simulink model "Thesis_MMC_WF_Modify"  (R2023a)
settings: Solver=VariableStepAuto  StartTime=0.0  StopTime=16  RelTol=1e-3
InitFcn:
  | % TS %
  | Ts_Control=4e-05;
  | Ts_Power=2e-05;
  | %% Main Circuit %%
  | % AC Line %
  | Vnom_Sec=333000;
  | Vnom_Pri=400000;
  | Pnom=1.0e+09;
  | Fnom=60;
  | Psc=2.0e+10;
  | P_Ld1=2/3*1e+09;
  | R_Startup=400;
  | Rxfo=0.003;
  | Lxfo=0.12;
  | P_Ld2=500e+03;
  | % MMC Parameter %
  | Larm_pu=0.15;
  | Rarm_pu=Larm_pu/100;
  | Zbase= Vnom_Sec^2/Pnom;
  | Larm=Larm_pu*(Zbase/(2*pi*Fnom));
  | Rarm=Rarm_pu*Zbase;
  | C_PM=1.758e-3;
  | w=2*pi*Fnom;
  | wc2=(2*w)^2;
  | Cfilter=1/(Larm*wc2);
  | Rfilter=1/(Cfilter*w)*30;
  | Topen_Filter=1e6;
  | K_V_dc=600000;
  | n=36;
  | Rg=100;
  | Cg=5e-08;
  | % HVDC Parameter %
  | R_cable=0.5;
  | L_cable=0.015;
  | %% Controller Parameter %%
  | % PLL %
  | Fn_filter=1000;
  | Zeta_filter=1;
  | % Active Power Regulator %
  | Kp_Preg=1/6;
  | Ki_Preg=1;
  | Limits_Preg=[0.8 1.2];
  | set_param('Thesis_MMC_WF_Modify/Controller/Active Power Regulator/Sum1','SampleTime','Ts_Control')
  | set_param('Thesis_MMC_WF_Modify/Controller/Active Power Regulator/Saturation','SampleTime','Ts_Control')
  | % Reactive Power Regulator %
  | Kp_Qreg=1/6;
  | Ki_Qreg=1;
  | Limits_Qreg=[-0.25 0.25];
  | set_param('Thesis_MMC_WF_Modify/Controller/Reactive Power Regulartor/Sum1','SampleTime','Ts_Control')
  | % Discrete Mean %
  | K1=3.2312e-30;
  | K2=-1.1369e-16;
  | Delay=0.02;
  | Vint=0;
  | Delay1=0.02004;
  | % DC Voltage Regulator %
  | Kp_VDCreg=4;
  | Ki_VDCreg=100;
  | Limits_VDCreg=[-2 2];
  | set_param('Thesis_MMC_WF_Modify/Controller/DC Voltage Regulator/Sum1','SampleTime','Ts_Control')
  | ... (+46 lines)
undefined symbols (not defined in the file): D1, Delta, Delta1, DiscIntNeverNeededParam, Lagging, Vnom_dc
libraries: spsSeriesRLCBranchLib x54, spsIGBTLib x24, spsBreakerLib x13, spsVoltageMeasurementLib x11, spsThreePhaseBreakerLib x11, spsThreePhaseVIMeasurementLib x9, spsIdealSwitchLib x8, simulink x7, spsDiscreteVariableTimeDelayLib x7, spsCurrentMeasurementLib x6, spsGroundLib x6, spsSecondOrderFilterLib x6
(part 2 of 3)

== system Thesis_MMC_WF_Modify/Inverter1 ==
  Constant6 : Constant  Value=480000/2  SampleTime=Ts_Power
  Controlled Voltage Source : spsControlledVoltageSourceLib/Controlled Voltage Source  Initialize=off  Source_Type=DC  Amplitude=0  Phase=0  Frequency=0  Measurements=None
  Controlled Voltage Source4 : spsControlledVoltageSourceLib/Controlled Voltage Source  Initialize=off  Source_Type=DC  Amplitude=0  Phase=0  Frequency=0  Measurements=None
  Ground : spsGroundLib/Ground  LConnTagsString=a
  Ideal Switch : spsIdealSwitchLib/Ideal Switch  Ron=0.001  Lon=0  IC=0  Rs=1e6  Cs=inf  Measurements=off
  Ideal Switch1 : spsIdealSwitchLib/Ideal Switch  Ron=0.001  Lon=0  IC=0  Rs=1e6  Cs=inf  Measurements=off
  Series RLC Branch : spsSeriesRLCBranchLib/Series RLC Branch  LConnTagsString=__new0  RConnTagsString=__new0  BranchType=RC  Resistance=1e-3  Inductance=1e-3  SetiL0=off  InitialCurrent=0  Capacitance=C_PM/n*3  Setx0=off  InitialVoltage=0  Measurements=None
  Series RLC Branch1 : spsSeriesRLCBranchLib/Series RLC Branch  LConnTagsString=__new0  RConnTagsString=__new0  BranchType=RC  Resistance=1e-3  Inductance=1e-3  SetiL0=off  InitialCurrent=0  Capacitance=C_PM/n*3  Setx0=off  InitialVoltage=0  Measurements=None
  Series RLC Branch2 : spsSeriesRLCBranchLib/Series RLC Branch  LConnTagsString=__new0  RConnTagsString=__new0  BranchType=R  Resistance=1e-3  Inductance=1e-3  SetiL0=off  InitialCurrent=0  Capacitance=1e-6  Setx0=off  InitialVoltage=0  Measurements=None
  Series RLC Branch3 : spsSeriesRLCBranchLib/Series RLC Branch  LConnTagsString=__new0  RConnTagsString=__new0  BranchType=R  Resistance=1e-3  Inductance=1e-3  SetiL0=off  InitialCurrent=0  Capacitance=1e-6  Setx0=off  InitialVoltage=0  Measurements=None
  Series RLC Branch5 : spsSeriesRLCBranchLib/Series RLC Branch  LConnTagsString=__new0  RConnTagsString=__new0  BranchType=RL  Resistance=1e-2  Inductance=1e-4  SetiL0=off  InitialCurrent=0  Capacitance=1e-6  Setx0=off  InitialVoltage=0  Measurements=None
  Series RLC Branch6 : spsSeriesRLCBranchLib/Series RLC Branch  LConnTagsString=__new0  RConnTagsString=__new0  BranchType=RL  Resistance=1e-2  Inductance=1e-4  SetiL0=off  InitialCurrent=0  Capacitance=1e-6  Setx0=off  InitialVoltage=0  Measurements=None
  Voltage Measurement1 : spsVoltageMeasurementLib/Voltage Measurement  PhasorSimulation=off  OutputType=Complex  PSBequivalent=0
  1 : PMIOPort  Side=Left
  2 : PMIOPort  Port=2  Side=Left
  tag scope: Vdc2=global
  wires:
  Constant6/1 -> Controlled Voltage Source/1, Controlled Voltage Source4/1
  [Inverter1_On] -> Ideal Switch/1, Ideal Switch1/1
  Voltage Measurement1/1 -> [Vdc2]
  connections:
  2/RConn1 -- Voltage Measurement1/LConn2 -- Series RLC Branch3/LConn1 -- Series RLC Branch1/RConn1
  Ideal Switch1/RConn1 -- Series RLC Branch6/RConn1
  Controlled Voltage Source4/RConn1 -- Controlled Voltage Source/LConn1 -- Series RLC Branch1/LConn1 -- Series RLC Branch/RConn1 -- Ground/LConn1
  Ideal Switch/RConn1 -- Series RLC Branch5/LConn1
  1/RConn1 -- Voltage Measurement1/LConn1 -- Series RLC Branch2/LConn1 -- Series RLC Branch/LConn1
  Series RLC Branch3/RConn1 -- Ideal Switch1/LConn1
  Series RLC Branch2/RConn1 -- Ideal Switch/LConn1
  Controlled Voltage Source/RConn1 -- Series RLC Branch5/RConn1
  Controlled Voltage Source4/LConn1 -- Series RLC Branch6/LConn1

== system Thesis_MMC_WF_Modify/Inverter2 ==
  Constant6 : Constant  Value=640000/2  SampleTime=Ts_Power
  Controlled Voltage Source : spsControlledVoltageSourceLib/Controlled Voltage Source  Initialize=off  Source_Type=DC  Amplitude=0  Phase=0  Frequency=0  Measurements=None
  Controlled Voltage Source4 : spsControlledVoltageSourceLib/Controlled Voltage Source  Initialize=off  Source_Type=DC  Amplitude=0  Phase=0  Frequency=0  Measurements=None
  Ground : spsGroundLib/Ground  LConnTagsString=a
  Ideal Switch : spsIdealSwitchLib/Ideal Switch  Ron=0.001  Lon=0  IC=0  Rs=1e6  Cs=inf  Measurements=off
  Ideal Switch1 : spsIdealSwitchLib/Ideal Switch  Ron=0.001  Lon=0  IC=0  Rs=1e6  Cs=inf  Measurements=off
  Series RLC Branch : spsSeriesRLCBranchLib/Series RLC Branch  LConnTagsString=__new0  RConnTagsString=__new0  BranchType=RC  Resistance=1e-3  Inductance=1e-3  SetiL0=off  InitialCurrent=0  Capacitance=C_PM/n*3  Setx0=off  InitialVoltage=0  Measurements=None
  Series RLC Branch1 : spsSeriesRLCBranchLib/Series RLC Branch  LConnTagsString=__new0  RConnTagsString=__new0  BranchType=RC  Resistance=1e-3  Inductance=1e-3  SetiL0=off  InitialCurrent=0  Capacitance=C_PM/n*3  Setx0=off  InitialVoltage=0  Measurements=None
  Series RLC Branch2 : spsSeriesRLCBranchLib/Series RLC Branch  LConnTagsString=__new0  RConnTagsString=__new0  BranchType=R  Resistance=1e-3  Inductance=1e-3  SetiL0=off  InitialCurrent=0  Capacitance=1e-6  Setx0=off  InitialVoltage=0  Measurements=None
  Series RLC Branch3 : spsSeriesRLCBranchLib/Series RLC Branch  LConnTagsString=__new0  RConnTagsString=__new0  BranchType=R  Resistance=1e-3  Inductance=1e-3  SetiL0=off  InitialCurrent=0  Capacitance=1e-6  Setx0=off  InitialVoltage=0  Measurements=None
  Series RLC Branch5 : spsSeriesRLCBranchLib/Series RLC Branch  LConnTagsString=__new0  RConnTagsString=__new0  BranchType=RL  Resistance=1e-2  Inductance=1e-4  SetiL0=off  InitialCurrent=0  Capacitance=1e-6  Setx0=off  InitialVoltage=0  Measurements=None
  Series RLC Branch6 : spsSeriesRLCBranchLib/Series RLC Branch  LConnTagsString=__new0  RConnTagsString=__new0  BranchType=RL  Resistance=1e-2  Inductance=1e-4  SetiL0=off  InitialCurrent=0  Capacitance=1e-6  Setx0=off  InitialVoltage=0  Measurements=None
  Voltage Measurement1 : spsVoltageMeasurementLib/Voltage Measurement  PhasorSimulation=off  OutputType=Complex  PSBequivalent=0
  1 : PMIOPort  Side=Left
  2 : PMIOPort  Port=2  Side=Left
  tag scope: Vdc4=global
  wires:
  Constant6/1 -> Controlled Voltage Source/1, Controlled Voltage Source4/1
  [Inverter2_On] -> Ideal Switch/1, Ideal Switch1/1
  Voltage Measurement1/1 -> [Vdc4]
  connections:
  2/RConn1 -- Voltage Measurement1/LConn2 -- Series RLC Branch3/LConn1 -- Series RLC Branch1/RConn1
  Ideal Switch1/RConn1 -- Series RLC Branch6/RConn1
  Series RLC Branch/RConn1 -- Ground/LConn1 -- Controlled Voltage Source/LConn1 -- Controlled Voltage Source4/RConn1 -- Series RLC Branch1/LConn1
  Ideal Switch/RConn1 -- Series RLC Branch5/LConn1
  1/RConn1 -- Voltage Measurement1/LConn1 -- Series RLC Branch2/LConn1 -- Series RLC Branch/LConn1
  Series RLC Branch3/RConn1 -- Ideal Switch1/LConn1
  Series RLC Branch2/RConn1 -- Ideal Switch/LConn1
  Controlled Voltage Source/RConn1 -- Series RLC Branch5/RConn1
  Controlled Voltage Source4/LConn1 -- Series RLC Branch6/LConn1

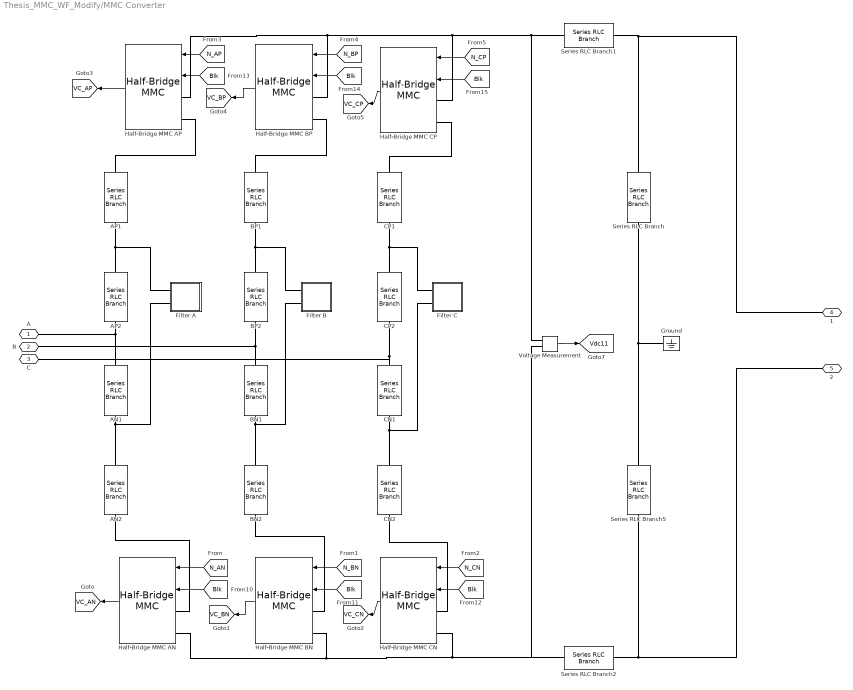
== system Thesis_MMC_WF_Modify/MMC Converter ==
  AN1 : spsSeriesRLCBranchLib/Series RLC Branch  LConnTagsString=__new0  RConnTagsString=__new0  BranchType=RL  Resistance=Rarm/2  Inductance=Larm/2  SetiL0=off  InitialCurrent=0  Capacitance=1e-6  Setx0=off  InitialVoltage=0  Measurements=None
  AN2 : spsSeriesRLCBranchLib/Series RLC Branch  LConnTagsString=__new0  RConnTagsString=__new0  BranchType=RL  Resistance=Rarm/2  Inductance=Larm/2  SetiL0=off  InitialCurrent=0  Capacitance=1e-6  Setx0=off  InitialVoltage=0  Measurements=None
  AP1 : spsSeriesRLCBranchLib/Series RLC Branch  LConnTagsString=__new0  RConnTagsString=__new0  BranchType=RL  Resistance=Rarm/2  Inductance=Larm/2  SetiL0=off  InitialCurrent=0  Capacitance=1e-6  Setx0=off  InitialVoltage=0  Measurements=None
  AP2 : spsSeriesRLCBranchLib/Series RLC Branch  LConnTagsString=__new0  RConnTagsString=__new0  BranchType=RL  Resistance=Rarm/2  Inductance=Larm/2  SetiL0=off  InitialCurrent=0  Capacitance=1e-6  Setx0=off  InitialVoltage=0  Measurements=None
  BN1 : spsSeriesRLCBranchLib/Series RLC Branch  LConnTagsString=__new0  RConnTagsString=__new0  BranchType=RL  Resistance=Rarm/2  Inductance=Larm/2  SetiL0=off  InitialCurrent=0  Capacitance=1e-6  Setx0=off  InitialVoltage=0  Measurements=None
  BN2 : spsSeriesRLCBranchLib/Series RLC Branch  LConnTagsString=__new0  RConnTagsString=__new0  BranchType=RL  Resistance=Rarm/2  Inductance=Larm/2  SetiL0=off  InitialCurrent=0  Capacitance=1e-6  Setx0=off  InitialVoltage=0  Measurements=None
  BP1 : spsSeriesRLCBranchLib/Series RLC Branch  LConnTagsString=__new0  RConnTagsString=__new0  BranchType=RL  Resistance=Rarm/2  Inductance=Larm/2  SetiL0=off  InitialCurrent=0  Capacitance=1e-6  Setx0=off  InitialVoltage=0  Measurements=None
  BP2 : spsSeriesRLCBranchLib/Series RLC Branch  LConnTagsString=__new0  RConnTagsString=__new0  BranchType=RL  Resistance=Rarm/2  Inductance=Larm/2  SetiL0=off  InitialCurrent=0  Capacitance=1e-6  Setx0=off  InitialVoltage=0  Measurements=None
  CN1 : spsSeriesRLCBranchLib/Series RLC Branch  LConnTagsString=__new0  RConnTagsString=__new0  BranchType=RL  Resistance=Rarm/2  Inductance=Larm/2  SetiL0=off  InitialCurrent=0  Capacitance=1e-6  Setx0=off  InitialVoltage=0  Measurements=None
  CN2 : spsSeriesRLCBranchLib/Series RLC Branch  LConnTagsString=__new0  RConnTagsString=__new0  BranchType=RL  Resistance=Rarm/2  Inductance=Larm/2  SetiL0=off  InitialCurrent=0  Capacitance=1e-6  Setx0=off  InitialVoltage=0  Measurements=None
  CP1 : spsSeriesRLCBranchLib/Series RLC Branch  LConnTagsString=__new0  RConnTagsString=__new0  BranchType=RL  Resistance=Rarm/2  Inductance=Larm/2  SetiL0=off  InitialCurrent=0  Capacitance=1e-6  Setx0=off  InitialVoltage=0  Measurements=None
  CP2 : spsSeriesRLCBranchLib/Series RLC Branch  LConnTagsString=__new0  RConnTagsString=__new0  BranchType=RL  Resistance=Rarm/2  Inductance=Larm/2  SetiL0=off  InitialCurrent=0  Capacitance=1e-6  Setx0=off  InitialVoltage=0  Measurements=None
  Filter A : Subsystem
  Filter B : Subsystem
  Filter C : Subsystem
  Ground : spsGroundLib/Ground  LConnTagsString=a
  Half-Bridge MMC AN : spsHalfBridgeMMCLib/Half-Bridge MMC  ModelType=Aggregate model  n=36  C=C_PM  Vc_Initial=0  Ron=1e-3  Rs=1e6  Cs=inf  Ron_Diode=1e-3  Rs_Diode=1e6  Cs_Diode=inf  Vf_Diode=1e-3  Rs_CurrentSource=inf  Ts=Ts_Power
      settings: LibrarySourceBlock=sps_lib/Power Electronics/Half-Bridge MMC
  Half-Bridge MMC AP : spsHalfBridgeMMCLib/Half-Bridge MMC  ModelType=Aggregate model  n=36  C=C_PM  Vc_Initial=0  Ron=1e-3  Rs=1e6  Cs=inf  Ron_Diode=1e-3  Rs_Diode=1e6  Cs_Diode=inf  Vf_Diode=1e-3  Rs_CurrentSource=inf  Ts=Ts_Power
      settings: LibrarySourceBlock=sps_lib/Power Electronics/Half-Bridge MMC
  Half-Bridge MMC BN : spsHalfBridgeMMCLib/Half-Bridge MMC  ModelType=Aggregate model  n=36  C=C_PM  Vc_Initial=0  Ron=1e-3  Rs=1e6  Cs=inf  Ron_Diode=1e-3  Rs_Diode=1e6  Cs_Diode=inf  Vf_Diode=1e-3  Rs_CurrentSource=inf  Ts=Ts_Power
      settings: LibrarySourceBlock=sps_lib/Power Electronics/Half-Bridge MMC
  Half-Bridge MMC BP : spsHalfBridgeMMCLib/Half-Bridge MMC  ModelType=Aggregate model  n=36  C=C_PM  Vc_Initial=0  Ron=1e-3  Rs=1e6  Cs=inf  Ron_Diode=1e-3  Rs_Diode=1e6  Cs_Diode=inf  Vf_Diode=1e-3  Rs_CurrentSource=inf  Ts=Ts_Power
      settings: LibrarySourceBlock=sps_lib/Power Electronics/Half-Bridge MMC
  Half-Bridge MMC CN : spsHalfBridgeMMCLib/Half-Bridge MMC  ModelType=Aggregate model  n=36  C=C_PM  Vc_Initial=0  Ron=1e-3  Rs=1e6  Cs=inf  Ron_Diode=1e-3  Rs_Diode=1e6  Cs_Diode=inf  Vf_Diode=1e-3  Rs_CurrentSource=inf  Ts=10e-6
      settings: LibrarySourceBlock=sps_lib/Power Electronics/Half-Bridge MMC
  Half-Bridge MMC CP : spsHalfBridgeMMCLib/Half-Bridge MMC  ModelType=Aggregate model  n=36  C=C_PM  Vc_Initial=0  Ron=1e-3  Rs=1e6  Cs=inf  Ron_Diode=1e-3  Rs_Diode=1e6  Cs_Diode=inf  Vf_Diode=1e-3  Rs_CurrentSource=inf  Ts=Ts_Power
      settings: LibrarySourceBlock=sps_lib/Power Electronics/Half-Bridge MMC
  Series RLC Branch : spsSeriesRLCBranchLib/Series RLC Branch  LConnTagsString=__new0  RConnTagsString=__new0  BranchType=RC  Resistance=Rg  Inductance=1e-3  SetiL0=off  InitialCurrent=0  Capacitance=Cg  Setx0=off  InitialVoltage=0  Measurements=None
  Series RLC Branch1 : spsSeriesRLCBranchLib/Series RLC Branch  LConnTagsString=__new0  RConnTagsString=__new0  BranchType=L  Resistance=1  Inductance=9e-1  SetiL0=off  InitialCurrent=0  Capacitance=1e-6  Setx0=off  InitialVoltage=0  Measurements=None
  Series RLC Branch2 : spsSeriesRLCBranchLib/Series RLC Branch  LConnTagsString=__new0  RConnTagsString=__new0  BranchType=L  Resistance=1  Inductance=9e-1  SetiL0=off  InitialCurrent=0  Capacitance=1e-6  Setx0=off  InitialVoltage=0  Measurements=None
  Series RLC Branch5 : spsSeriesRLCBranchLib/Series RLC Branch  LConnTagsString=__new0  RConnTagsString=__new0  BranchType=RC  Resistance=Rg  Inductance=1e-3  SetiL0=off  InitialCurrent=0  Capacitance=Cg  Setx0=off  InitialVoltage=0  Measurements=None
  Voltage Measurement : spsVoltageMeasurementLib/Voltage Measurement  PhasorSimulation=off  OutputType=Complex  PSBequivalent=0
  A : PMIOPort  Side=Left
  B : PMIOPort  Port=2  Side=Left
  C : PMIOPort  Port=3  Side=Left
  1 : PMIOPort  Port=4  Side=Right
  2 : PMIOPort  Port=5  Side=Right
  tag scope: VC_AN=global, VC_AP=global, VC_BN=global, VC_BP=global, VC_CN=global, VC_CP=global, Vdc11=global
  wires:
  Half-Bridge MMC CN/1 -> [VC_CN]
  [N_BN] -> Half-Bridge MMC BN/1
  [Blk] -> Half-Bridge MMC BN/2
  [Blk] -> Half-Bridge MMC CN/2
  [Blk] -> Half-Bridge MMC AN/2
  [Blk] -> Half-Bridge MMC AP/2
  [N_CN] -> Half-Bridge MMC CN/1
  [N_BP] -> Half-Bridge MMC BP/1
  Half-Bridge MMC BN/1 -> [VC_BN]
  Half-Bridge MMC CP/1 -> [VC_CP]
  Half-Bridge MMC BP/1 -> [VC_BP]
  [Blk] -> Half-Bridge MMC BP/2
  [N_AN] -> Half-Bridge MMC AN/1
  [N_AP] -> Half-Bridge MMC AP/1
  [N_CP] -> Half-Bridge MMC CP/1
  [Blk] -> Half-Bridge MMC CP/2
  Half-Bridge MMC AP/1 -> [VC_AP]
  Half-Bridge MMC AN/1 -> [VC_AN]
  Voltage Measurement/1 -> [Vdc11]
  connections:
  2/RConn1 -- Series RLC Branch2/RConn1 -- Series RLC Branch5/RConn1
  CN1/LConn1 -- Filter C/LConn2 -- CN2/RConn1
  BN1/RConn1 -- B/RConn1 -- BP2/RConn1
  CP2/LConn1 -- Filter C/LConn1 -- CP1/RConn1
  CP2/RConn1 -- C/RConn1 -- CN1/RConn1
  Series RLC Branch5/LConn1 -- Ground/LConn1 -- Series RLC Branch/RConn1
  BN1/LConn1 -- Filter B/LConn2 -- BN2/RConn1
  Voltage Measurement/LConn1 -- Series RLC Branch1/LConn1 -- Half-Bridge MMC CP/LConn1 -- Half-Bridge MMC BP/LConn1 -- Half-Bridge MMC AP/LConn1
  AN1/LConn1 -- AN2/RConn1 -- Filter A/LConn2
  AP2/RConn1 -- A/RConn1 -- AN1/RConn1
  BP2/LConn1 -- Filter B/LConn1 -- BP1/RConn1
  AP1/RConn1 -- AP2/LConn1 -- Filter A/LConn1
  AN2/LConn1 -- Half-Bridge MMC AN/LConn1
  AP1/LConn1 -- Half-Bridge MMC AP/LConn2
  BN2/LConn1 -- Half-Bridge MMC BN/LConn1
  BP1/LConn1 -- Half-Bridge MMC BP/LConn2
  Half-Bridge MMC CN/LConn1 -- CN2/LConn1
  CP1/LConn1 -- Half-Bridge MMC CP/LConn2
  Half-Bridge MMC CN/LConn2 -- Series RLC Branch2/LConn1 -- Voltage Measurement/LConn2 -- Half-Bridge MMC BN/LConn2 -- Half-Bridge MMC AN/LConn2
  1/RConn1 -- Series RLC Branch1/RConn1 -- Series RLC Branch/LConn1

== system Thesis_MMC_WF_Modify/Prim1 ==
  Three-Phase V-I Measurement : spsThreePhaseVIMeasurementLib/Three-Phase V-I Measurement  VoltageMeasurement=phase-to-ground  SetLabelV=off  LabelV=Vabc  Vpu=off  VpuLL=off  CurrentMeasurement=yes  SetLabelI=off  LabelI=Iabc  Ipu=off  Pbase=100e6  Vbase=500e3  OutputType=Complex  PhasorSimulation=off  PSBequivalent=0
  A : PMIOPort  Side=Left
  B : PMIOPort  Port=2  Side=Left
  a : PMIOPort  Port=3  Side=Right
  b : PMIOPort  Port=4  Side=Right
  C : PMIOPort  Port=5  Side=Left
  c : PMIOPort  Port=6  Side=Right
  tag scope: Iprim1=global, Vprim1=global
  wires:
  Three-Phase V-I Measurement/2 -> [Iprim1]
  Three-Phase V-I Measurement/1 -> [Vprim1]
  connections:
  Three-Phase V-I Measurement/LConn1 -- A/RConn1
  Three-Phase V-I Measurement/RConn2 -- b/RConn1
  Three-Phase V-I Measurement/LConn2 -- B/RConn1
  Three-Phase V-I Measurement/RConn3 -- c/RConn1
  Three-Phase V-I Measurement/RConn1 -- a/RConn1
  Three-Phase V-I Measurement/LConn3 -- C/RConn1

== system Thesis_MMC_WF_Modify/Prim2 ==
  Three-Phase V-I Measurement : spsThreePhaseVIMeasurementLib/Three-Phase V-I Measurement  VoltageMeasurement=phase-to-ground  SetLabelV=off  LabelV=Vabc  Vpu=off  VpuLL=off  CurrentMeasurement=yes  SetLabelI=off  LabelI=Iabc  Ipu=off  Pbase=100e6  Vbase=500e3  OutputType=Complex  PhasorSimulation=off  PSBequivalent=0
  A : PMIOPort  Side=Left
  B : PMIOPort  Port=2  Side=Left
  a : PMIOPort  Port=3  Side=Right
  b : PMIOPort  Port=4  Side=Right
  C : PMIOPort  Port=5  Side=Left
  c : PMIOPort  Port=6  Side=Right
  tag scope: Iprim2=global, Vprim2=global
  wires:
  Three-Phase V-I Measurement/2 -> [Iprim2]
  Three-Phase V-I Measurement/1 -> [Vprim2]
  connections:
  Three-Phase V-I Measurement/LConn1 -- A/RConn1
  Three-Phase V-I Measurement/RConn2 -- b/RConn1
  Three-Phase V-I Measurement/LConn2 -- B/RConn1
  Three-Phase V-I Measurement/RConn3 -- c/RConn1
  Three-Phase V-I Measurement/RConn1 -- a/RConn1
  Three-Phase V-I Measurement/LConn3 -- C/RConn1

== system Thesis_MMC_WF_Modify/Prim3 ==
  Three-Phase V-I Measurement : spsThreePhaseVIMeasurementLib/Three-Phase V-I Measurement  VoltageMeasurement=phase-to-ground  SetLabelV=off  LabelV=Vabc  Vpu=off  VpuLL=off  CurrentMeasurement=yes  SetLabelI=off  LabelI=Iabc  Ipu=off  Pbase=100e6  Vbase=500e3  OutputType=Complex  PhasorSimulation=off  PSBequivalent=0
  A : PMIOPort  Side=Left
  B : PMIOPort  Port=2  Side=Left
  a : PMIOPort  Port=3  Side=Right
  b : PMIOPort  Port=4  Side=Right
  C : PMIOPort  Port=5  Side=Left
  c : PMIOPort  Port=6  Side=Right
  tag scope: Iprim3=global, Vprim3=global
  wires:
  Three-Phase V-I Measurement/2 -> [Iprim3]
  Three-Phase V-I Measurement/1 -> [Vprim3]
  connections:
  Three-Phase V-I Measurement/LConn1 -- A/RConn1
  Three-Phase V-I Measurement/RConn2 -- b/RConn1
  Three-Phase V-I Measurement/LConn2 -- B/RConn1
  Three-Phase V-I Measurement/RConn3 -- c/RConn1
  Three-Phase V-I Measurement/RConn1 -- a/RConn1
  Three-Phase V-I Measurement/LConn3 -- C/RConn1

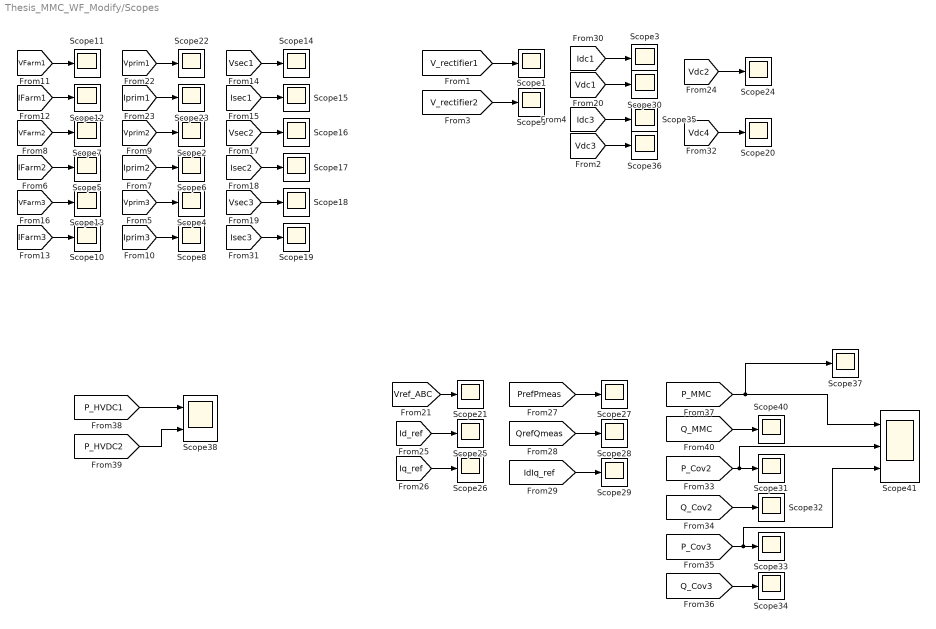
== system Thesis_MMC_WF_Modify/Scopes ==
  Scope{1..37,40} (38 alike) : Scope
  Scope38 : Scope  NumInputPorts=2
  Scope41 : Scope  NumInputPorts=3
  wires:
  [Vref_ABC] -> Scope21/1
  [Vprim1] -> Scope22/1
  [Isec1] -> Scope15/1
  [Iprim1] -> Scope23/1
  [Vsec1] -> Scope14/1
  [Vdc2] -> Scope24/1
  [Id_ref] -> Scope25/1
  [Iq_ref] -> Scope26/1
  [PrefPmeas] -> Scope27/1
  [QrefQmeas] -> Scope28/1
  [IdIq_ref] -> Scope29/1
  [Idc1] -> Scope3/1
  [V_rectifier2] -> Scope9/1
  [V_rectifier1] -> Scope1/1
  [Vdc3] -> Scope36/1
  [Idc3] -> Scope35/1
  [IFarm2] -> Scope5/1
  [VFarm2] -> Scope7/1
  [Vprim3] -> Scope4/1
  [Iprim2] -> Scope6/1
  [VFarm1] -> Scope11/1
  [IFarm1] -> Scope12/1
  [Vdc1] -> Scope30/1
  [Vprim2] -> Scope2/1
  [Iprim3] -> Scope8/1
  [IFarm3] -> Scope10/1
  [VFarm3] -> Scope13/1
  [Isec2] -> Scope17/1
  [Vsec2] -> Scope16/1
  [Isec3] -> Scope19/1
  [Vsec3] -> Scope18/1
  [Vdc4] -> Scope20/1
  [Q_Cov2] -> Scope32/1
  [P_Cov2] -> Scope41/2, Scope31/1
  [Q_Cov3] -> Scope34/1
  [P_Cov3] -> Scope41/3, Scope33/1
  [P_MMC] -> Scope41/1, Scope37/1
  [P_HVDC1] -> Scope38/1
  [P_HVDC2] -> Scope38/2
  [Q_MMC] -> Scope40/1

== system Thesis_MMC_WF_Modify/Sec1 ==
  Three-Phase V-I Measurement : spsThreePhaseVIMeasurementLib/Three-Phase V-I Measurement  VoltageMeasurement=phase-to-ground  SetLabelV=off  LabelV=Vabc  Vpu=off  VpuLL=off  CurrentMeasurement=yes  SetLabelI=off  LabelI=Iabc  Ipu=off  Pbase=100e6  Vbase=500e3  OutputType=Complex  PhasorSimulation=off  PSBequivalent=0
  A : PMIOPort  Side=Left
  B : PMIOPort  Port=2  Side=Left
  a : PMIOPort  Port=3  Side=Right
  b : PMIOPort  Port=4  Side=Right
  C : PMIOPort  Port=5  Side=Left
  c : PMIOPort  Port=6  Side=Right
  tag scope: Isec1=global, Vsec1=global
  wires:
  Three-Phase V-I Measurement/2 -> [Isec1]
  Three-Phase V-I Measurement/1 -> [Vsec1]
  connections:
  Three-Phase V-I Measurement/LConn1 -- A/RConn1
  Three-Phase V-I Measurement/RConn2 -- b/RConn1
  Three-Phase V-I Measurement/LConn2 -- B/RConn1
  Three-Phase V-I Measurement/RConn3 -- c/RConn1
  Three-Phase V-I Measurement/RConn1 -- a/RConn1
  Three-Phase V-I Measurement/LConn3 -- C/RConn1

== system Thesis_MMC_WF_Modify/Controller/Active Power Regulator ==
  Pmeas : Inport
  Pref : Inport  Port=2
  on : Inport  Port=3
  Constant : Constant  Value=Ki_Preg  SampleTime=Ts_Control
  Constant1 : Constant  Value=Kp_Preg  SampleTime=Ts_Control
  Constant2 : Constant  Value=Vnom_dc  SampleTime=Ts_Control
  Discrete-Time Integrator : DiscreteIntegrator  InitialCondition=1  SampleTime=Ts_Control  LimitOutput=on  UpperSaturationLimit=Limits_Preg(2)  LowerSaturationLimit=Limits_Preg(1)  ICPrevOutput=DiscIntNeverNeededParam  ICPrevScaledInput=DiscIntNeverNeededParam
  Product : Product
  Product1 : Product
  Product2 : Product
  Saturation : Saturate  UpperLimit=Limits_Preg(2)  LowerLimit=Limits_Preg(1)  SampleTime=Ts_Control
  Sum : Sum  Inputs=|+-
  Sum1 : Sum  SampleTime=Ts_Control
  Switch : Switch  Criteria=u2 ~= 0  Threshold=0.5  SaturateOnIntegerOverflow=off  InputSameDT=off
  Zero-Order Hold : ZeroOrderHold  SampleTime=Ts_Control
  Vdc_ref : Outport
  wires:
  Pmeas/1 -> Switch/1
  on/1 -> Switch/2
  Switch/1 -> Sum/1
  Pref/1 -> Switch/3, Sum/2
  Sum/1 -> Product1/2, Product/2
  Constant/1 -> Product1/1
  Constant1/1 -> Product/1
  Product/1 -> Zero-Order Hold/1
  Product1/1 -> Discrete-Time Integrator/1
  Discrete-Time Integrator/1 -> Sum1/2
  Zero-Order Hold/1 -> Sum1/1
  Sum1/1 -> Saturation/1
  Saturation/1 -> Product2/1
  Constant2/1 -> Product2/2
  Product2/1 -> Vdc_ref/1

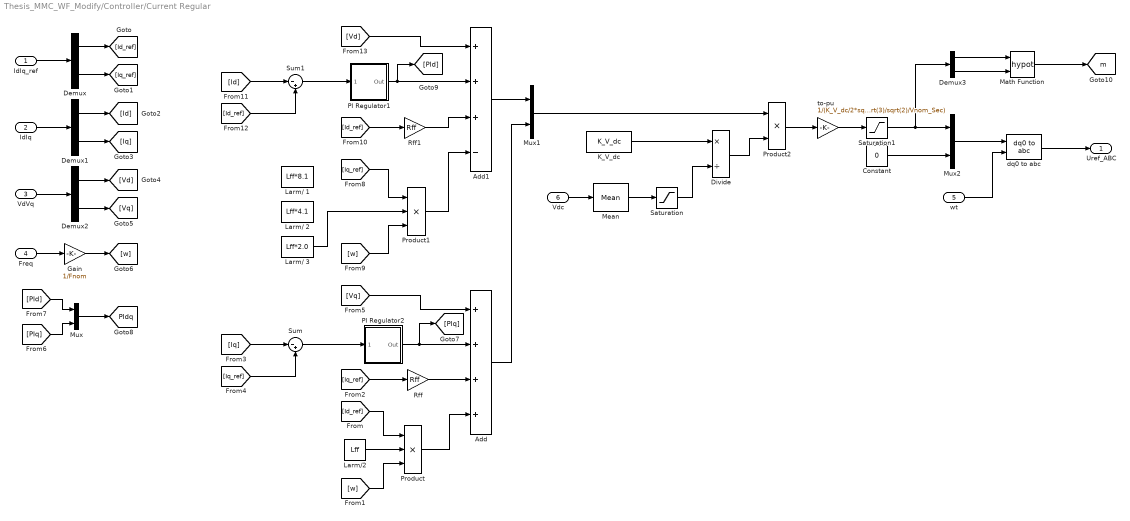
== system Thesis_MMC_WF_Modify/Controller/Current Regular ==
  IdIq_ref : Inport
  IdIq : Inport  Port=2
  VdVq : Inport  Port=3
  Freq : Inport  Port=4
  wt : Inport  Port=5
  Vdc : Inport  Port=6
  Add : Sum  Inputs=++++
  Add1 : Sum  Inputs=+++-
  Constant : Constant  Value=0
  Demux{,1..3} (4 alike) : Demux  Outputs=2
  Divide : Product  Inputs=*/
  Gain : Gain  Gain=1/Fnom
  K_V_dc : Constant  Value=K_V_dc  SampleTime=Ts_Control
  Larm/ 1 : Constant  Value=Lff*8.1  SampleTime=Ts_Control
  Larm/ 2 : Constant  Value=Lff*4.1  SampleTime=Ts_Control  LockScale=on
  Larm/ 3 : Constant  Value=Lff*2.0  SampleTime=Ts_Control
  Larm/2 : Constant  Value=Lff  SampleTime=Ts_Control
  Math Function : Math  Operator=hypot
  Mean : spsMeanLib/Mean  Freq=Fnom/3  Vinit=K_V_dc  Ts=Ts_Control
  Mux : Mux  Inputs=2
  Mux1 : Mux  Inputs=2
  Mux2 : Mux  Inputs=2
  PI Regulator1 : Subsystem
  PI Regulator2 : Subsystem
  Product : Product  Inputs=3
  Product1 : Product  Inputs=3
  Product2 : Product
  Rff : Gain  Gain=Rff
  Rff1 : Gain  Gain=Rff
  Saturation : Saturate  UpperLimit=500000  LowerLimit=450000
  Saturation1 : Saturate  UpperLimit=Limits_Ireg(2)  LowerLimit=Limits_Ireg(1)
  Sum : Sum  Inputs=|-+
  Sum1 : Sum  Inputs=|-+
  dq0 to abc : spsdq0toabcLib/dq0 to abc  Alignment=90 degrees behind phase A axis
  to-pu : Gain  Gain=1/(K_V_dc/2*sqrt(3)/sqrt(2)/Vnom_Sec)
  Uref_ABC : Outport
  tag scope: PIdq=global, m=global
  wires:
  IdIq_ref/1 -> Demux/1
  Demux/1 -> [Id_ref]
  Demux/2 -> [Iq_ref]
  IdIq/1 -> Demux1/1
  Demux1/1 -> [Id]
  Demux1/2 -> [Iq]
  VdVq/1 -> Demux2/1
  Demux2/1 -> [Vd]
  Demux2/2 -> [Vq]
  Freq/1 -> Gain/1
  Gain/1 -> [w]
  Larm/2/1 -> Product/2
  [w] -> Product/3
  [Id_ref] -> Product/1
  Product/1 -> Add/4
  Rff/1 -> Add/3
  [Iq_ref] -> Rff/1
  [Iq] -> Sum/1
  [Iq_ref] -> Sum/2
  [Vq] -> Add/1
  [PId] -> Mux/1
  [PIq] -> Mux/2
  Mux/1 -> [PIdq]
  [Iq_ref] -> Product1/1
  [w] -> Product1/3
  Product1/1 -> Add1/4
  [Id_ref] -> Rff1/1
  Rff1/1 -> Add1/3
  [Id] -> Sum1/1
  [Id_ref] -> Sum1/2
  [Vd] -> Add1/1
  Add1/1 -> Mux1/1
  Add/1 -> Mux1/2
  Divide/1 -> Product2/2
  Saturation/1 -> Divide/2
  Product2/1 -> to-pu/1
  to-pu/1 -> Saturation1/1
  Saturation1/1 -> Mux2/1, Demux3/1
  Constant/1 -> Mux2/2
  Mux2/1 -> dq0 to abc/1
  wt/1 -> dq0 to abc/2
  dq0 to abc/1 -> Uref_ABC/1
  Mean/1 -> Saturation/1
  Vdc/1 -> Mean/1
  Demux3/1 -> Math Function/1
  Demux3/2 -> Math Function/2
  Math Function/1 -> [m]
  Sum1/1 -> PI Regulator1/1(Error)
  PI Regulator1/1(Out) -> [PId], Add1/2
  Sum/1 -> PI Regulator2/1(Error)
  PI Regulator2/1(Out) -> [PIq], Add/2
  K_V_dc/1 -> Divide/1
  Mux1/1 -> Product2/1
  Larm/ 3/1 -> Product1/2

== system Thesis_MMC_WF_Modify/Controller/DC Voltage Regulator ==
  Vdc_meas : Inport
  Vdc_ref : Inport  Port=2
  on : Inport  Port=3
  Discrete-Time Integrator : DiscreteIntegrator  SampleTime=Ts_Control  LimitOutput=on  UpperSaturationLimit=Limits_VDCreg(2)  LowerSaturationLimit=Limits_VDCreg(1)  ICPrevOutput=DiscIntNeverNeededParam  ICPrevScaledInput=DiscIntNeverNeededParam
  Gain : Gain  Gain=K_V_dc  OutDataTypeStr=Inherit: Same as input  ParamDataTypeStr=Inherit: Same as input
  Ki1 : Constant  Value=Ki_VDCreg
  Kp1 : Constant  Value=Kp_VDCreg
  Product : Product  RndMeth=Zero
  Product1 : Product  RndMeth=Zero
  Saturation : Saturate  UpperLimit=Limits_VDCreg(2)  LowerLimit=Limits_VDCreg(1)  SampleTime=Ts_Control
  Sum : Sum  Inputs=|+-
  Sum1 : Sum  InputSameDT=on  SampleTime=Ts_Control
  Switch : Switch  Criteria=u2 ~= 0  Threshold=0.5  OutDataTypeStr=double  SaturateOnIntegerOverflow=off  InputSameDT=off
  Zero-Order Hold : ZeroOrderHold  SampleTime=Ts_Control
  Id_ref : Outport
  wires:
  Gain/1 -> Product/2, Product1/2
  Zero-Order Hold/1 -> Sum1/1
  Saturation/1 -> Id_ref/1
  Sum1/1 -> Saturation/1
  Ki1/1 -> Product1/1
  Product/1 -> Zero-Order Hold/1
  Switch/1 -> Sum/1
  Sum/1 -> Gain/1
  Vdc_meas/1 -> Switch/1
  Vdc_ref/1 -> Switch/3, Sum/2
  on/1 -> Switch/2
  Product1/1 -> Discrete-Time Integrator/1
  Discrete-Time Integrator/1 -> Sum1/2
  Kp1/1 -> Product/1

== system Thesis_MMC_WF_Modify/Controller/Fault Protection ==
  Blk_Con1_D : Step  Time=99999  SampleTime=Ts_Power
  Blk_Con1_D1 : Step  Time=10.5  Before=1  After=0  SampleTime=Ts_Power
  Blk_Con1_Y : Step  Time=99999  SampleTime=Ts_Power
  Blk_Con2_D : Step  Time=99999  SampleTime=Ts_Power
  Blk_Con2_Y : Step  Time=99999  SampleTime=Ts_Power
  Brk_ACAC : Step  Time=99999  SampleTime=Ts_Power
  Constant : Constant
  Constant1 : Constant
  Constant2 : Constant
  Logical Operator1 : Logic  Operator=OR  AllPortsSameDT=off  OutDataTypeStr=boolean
  Step : Step  Time=10.5  Before=1  After=0  SampleTime=Ts_Control
  tag scope: Blk_Fault1D=global, Blk_Fault1Y=global, Blk_Fault2D=global, Blk_Fault2Y=global, Brk3_Fault=global, Brk4_Fault=global, Brk_ACAC=global, Brk_WF1=global, Brk_WF2=global, Brk_WF3=global
  wires:
  Step/1 -> [Brk4_Fault]
  Logical Operator1/1 -> [Brk3_Fault]
  Blk_Con1_Y/1 -> [Blk_Fault1Y]
  Blk_Con1_D/1 -> [Blk_Fault1D]
  Blk_Con2_Y/1 -> [Blk_Fault2Y]
  Blk_Con2_D/1 -> [Blk_Fault2D]
  Brk_ACAC/1 -> [Brk_ACAC]
  Constant/1 -> [Brk_WF1]
  Constant1/1 -> [Brk_WF2]
  Constant2/1 -> [Brk_WF3]

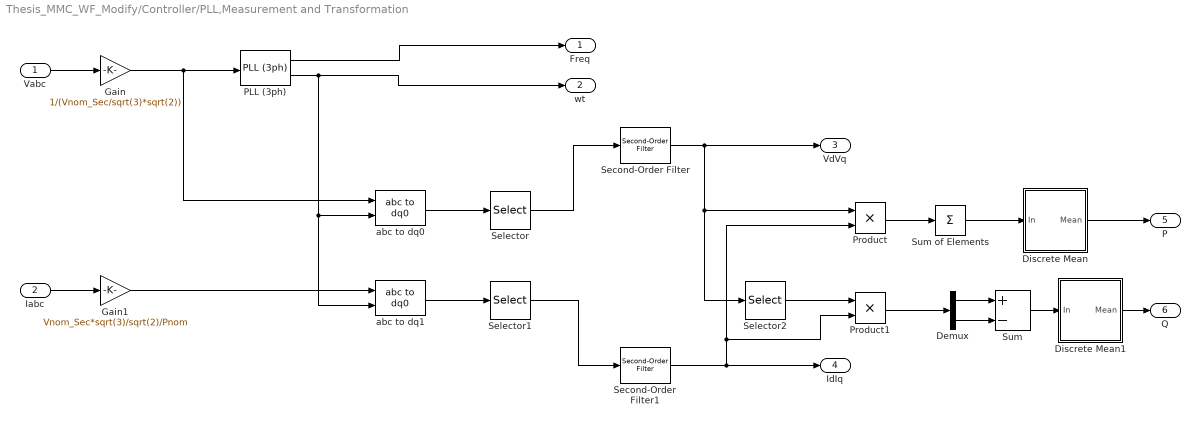
== system Thesis_MMC_WF_Modify/Controller/PLL,Measurement and Transformation ==
  Vabc : Inport
  Iabc : Inport  Port=2
  Demux : Demux  Outputs=2
  Discrete Mean : Subsystem
  Discrete Mean1 : Subsystem
  Gain : Gain  Gain=1/(Vnom_Sec/sqrt(3)*sqrt(2))
  Gain1 : Gain  Gain=Vnom_Sec*sqrt(3)/sqrt(2)/Pnom
  PLL (3ph) : spsPLL3phLib/PLL (3ph)  Fmin=0.9*Fnom  Par_Init=[0, Fnom]  ParK=[180, 3200, 1]  TcD=1e-4  MaxRateChangeFreq=12  FilterCutOffFreq=25  Ts=Ts_Control  AGC=on
  Product : Product
  Product1 : Product
  Second-Order Filter : spsSecondOrderFilterLib/Second-Order Filter  FilterType=Lowpass  Fo=Fn_filter  Zeta=Zeta_filter  Ts=Ts_Control  Initialize=off  Vac_Init="[0,  0,  60]"  Vdc_Init=0  PlotResponse=off  FreqRange=[0, 500, 1]
      settings: LibrarySourceBlock=|
      | sps_lib/Control/Filters/Second-Order
      | Filter
  Second-Order Filter1 : spsSecondOrderFilterLib/Second-Order Filter  FilterType=Lowpass  Fo=Fn_filter  Zeta=Zeta_filter  Ts=Ts_Control  Initialize=off  Vac_Init="[0,  0,  60]"  Vdc_Init=0  PlotResponse=off  FreqRange=[0, 500, 1]
      settings: LibrarySourceBlock=|
      | sps_lib/Control/Filters/Second-Order
      | Filter
  Selector : Selector  InputPortWidth=3  IndexOptions=Index vector (dialog)  Indices=[1 2]  OutputSizes=1
  Selector1 : Selector  InputPortWidth=3  IndexOptions=Index vector (dialog)  Indices=[1 2]  OutputSizes=1
  Selector2 : Selector  InputPortWidth=2  IndexOptions=Index vector (dialog)  Indices=[2 1]  OutputSizes=1
  Sum : Sum  Inputs=+-
  Sum of Elements : Sum  Inputs=1
  abc to dq0 : spsabctodq0Lib/abc to dq0  Alignment=90 degrees behind phase A axis
  abc to dq1 : spsabctodq0Lib/abc to dq0  Alignment=90 degrees behind phase A axis
  Freq : Outport
  wt : Outport  Port=2
  VdVq : Outport  Port=3
  IdIq : Outport  Port=4
  P : Outport  Port=5
  Q : Outport  Port=6
  wires:
  Vabc/1 -> Gain/1
  Iabc/1 -> Gain1/1
  Gain/1 -> abc to dq0/1, PLL (3ph)/1
  PLL (3ph)/1 -> Freq/1
  PLL (3ph)/2 -> abc to dq1/2, abc to dq0/2, wt/1
  Gain1/1 -> abc to dq1/1
  abc to dq0/1 -> Selector/1
  abc to dq1/1 -> Selector1/1
  Selector1/1 -> Second-Order Filter1/1
  Selector/1 -> Second-Order Filter/1
  Second-Order Filter/1 -> Product/1, Selector2/1, VdVq/1
  Second-Order Filter1/1 -> Product1/2, Product/2, IdIq/1
  Selector2/1 -> Product1/1
  Product/1 -> Sum of Elements/1
  Product1/1 -> Demux/1
  Demux/1 -> Sum/1
  Demux/2 -> Sum/2
  Sum of Elements/1 -> Discrete Mean/1(In)
  Discrete Mean/1(Mean) -> P/1
  Sum/1 -> Discrete Mean1/1(In)
  Discrete Mean1/1(Mean) -> Q/1

== system Thesis_MMC_WF_Modify/Controller/PLL,Measurement1 ==
  Vabc : Inport
  Iabc : Inport  Port=2
  Demux : Demux  Outputs=2
  Discrete Mean : Subsystem
  Discrete Mean1 : Subsystem
  Gain : Gain  Gain=1/(Vnom_Sec/sqrt(3)*sqrt(2))
  Gain1 : Gain  Gain=Vnom_Sec*sqrt(3)/sqrt(2)/Pnom
  PLL (3ph) : spsPLL3phLib/PLL (3ph)  Fmin=0.9*Fnom  Par_Init=[0, Fnom]  ParK=[180, 3200, 1]  TcD=1e-4  MaxRateChangeFreq=12  FilterCutOffFreq=25  Ts=Ts_Control  AGC=on
  Product : Product
  Product1 : Product
  Second-Order Filter : spsSecondOrderFilterLib/Second-Order Filter  FilterType=Lowpass  Fo=Fn_filter  Zeta=Zeta_filter  Ts=Ts_Control  Initialize=off  Vac_Init="[0,  0,  60]"  Vdc_Init=0  PlotResponse=off  FreqRange=[0, 500, 1]
      settings: LibrarySourceBlock=|
      | sps_lib/Control/Filters/Second-Order
      | Filter
  Second-Order Filter1 : spsSecondOrderFilterLib/Second-Order Filter  FilterType=Lowpass  Fo=Fn_filter  Zeta=Zeta_filter  Ts=Ts_Control  Initialize=off  Vac_Init="[0,  0,  60]"  Vdc_Init=0  PlotResponse=off  FreqRange=[0, 500, 1]
      settings: LibrarySourceBlock=|
      | sps_lib/Control/Filters/Second-Order
      | Filter
  Selector : Selector  InputPortWidth=3  IndexOptions=Index vector (dialog)  Indices=[1 2]  OutputSizes=1
  Selector1 : Selector  InputPortWidth=3  IndexOptions=Index vector (dialog)  Indices=[1 2]  OutputSizes=1
  Selector2 : Selector  InputPortWidth=2  IndexOptions=Index vector (dialog)  Indices=[2 1]  OutputSizes=1
  Sum : Sum  Inputs=+-
  Sum of Elements : Sum  Inputs=1
  Terminator : Terminator
  abc to dq0 : spsabctodq0Lib/abc to dq0  Alignment=90 degrees behind phase A axis
  abc to dq1 : spsabctodq0Lib/abc to dq0  Alignment=90 degrees behind phase A axis
  P : Outport
  Q : Outport  Port=2
  wires:
  Vabc/1 -> Gain/1
  Iabc/1 -> Gain1/1
  Gain/1 -> abc to dq0/1, PLL (3ph)/1
  PLL (3ph)/2 -> abc to dq1/2, abc to dq0/2
  Gain1/1 -> abc to dq1/1
  abc to dq0/1 -> Selector/1
  abc to dq1/1 -> Selector1/1
  Selector1/1 -> Second-Order Filter1/1
  Selector/1 -> Second-Order Filter/1
  Second-Order Filter/1 -> Product/1, Selector2/1
  Second-Order Filter1/1 -> Product1/2, Product/2
  Selector2/1 -> Product1/1
  Product/1 -> Sum of Elements/1
  Product1/1 -> Demux/1
  Demux/1 -> Sum/1
  Demux/2 -> Sum/2
  Sum of Elements/1 -> Discrete Mean/1(In)
  Discrete Mean/1(Mean) -> P/1
  Sum/1 -> Discrete Mean1/1(In)
  Discrete Mean1/1(Mean) -> Q/1
  PLL (3ph)/1 -> Terminator/1

== system Thesis_MMC_WF_Modify/Controller/PLL,Measurement2 ==
  Vabc : Inport
  Iabc : Inport  Port=2
  Demux : Demux  Outputs=2
  Discrete Mean : Subsystem
  Discrete Mean1 : Subsystem
  Gain : Gain  Gain=1/(Vnom_Sec/sqrt(3)*sqrt(2))
  Gain1 : Gain  Gain=Vnom_Sec*sqrt(3)/sqrt(2)/Pnom
  PLL (3ph) : spsPLL3phLib/PLL (3ph)  Fmin=0.9*Fnom  Par_Init=[0, Fnom]  ParK=[180, 3200, 1]  TcD=1e-4  MaxRateChangeFreq=12  FilterCutOffFreq=25  Ts=Ts_Control  AGC=on
  Product : Product
  Product1 : Product
  Second-Order Filter : spsSecondOrderFilterLib/Second-Order Filter  FilterType=Lowpass  Fo=Fn_filter  Zeta=Zeta_filter  Ts=Ts_Control  Initialize=off  Vac_Init="[0,  0,  60]"  Vdc_Init=0  PlotResponse=off  FreqRange=[0, 500, 1]
      settings: LibrarySourceBlock=|
      | sps_lib/Control/Filters/Second-Order
      | Filter
  Second-Order Filter1 : spsSecondOrderFilterLib/Second-Order Filter  FilterType=Lowpass  Fo=Fn_filter  Zeta=Zeta_filter  Ts=Ts_Control  Initialize=off  Vac_Init="[0,  0,  60]"  Vdc_Init=0  PlotResponse=off  FreqRange=[0, 500, 1]
      settings: LibrarySourceBlock=|
      | sps_lib/Control/Filters/Second-Order
      | Filter
  Selector : Selector  InputPortWidth=3  IndexOptions=Index vector (dialog)  Indices=[1 2]  OutputSizes=1
  Selector1 : Selector  InputPortWidth=3  IndexOptions=Index vector (dialog)  Indices=[1 2]  OutputSizes=1
  Selector2 : Selector  InputPortWidth=2  IndexOptions=Index vector (dialog)  Indices=[2 1]  OutputSizes=1
  Sum : Sum  Inputs=+-
  Sum of Elements : Sum  Inputs=1
  Terminator : Terminator
  abc to dq0 : spsabctodq0Lib/abc to dq0  Alignment=90 degrees behind phase A axis
  abc to dq1 : spsabctodq0Lib/abc to dq0  Alignment=90 degrees behind phase A axis
  P : Outport
  Q : Outport  Port=2
  wires:
  Vabc/1 -> Gain/1
  Iabc/1 -> Gain1/1
  Gain/1 -> abc to dq0/1, PLL (3ph)/1
  PLL (3ph)/2 -> abc to dq1/2, abc to dq0/2
  Gain1/1 -> abc to dq1/1
  abc to dq0/1 -> Selector/1
  abc to dq1/1 -> Selector1/1
  Selector1/1 -> Second-Order Filter1/1
  Selector/1 -> Second-Order Filter/1
  Second-Order Filter/1 -> Product/1, Selector2/1
  Second-Order Filter1/1 -> Product1/2, Product/2
  Selector2/1 -> Product1/1
  Product/1 -> Sum of Elements/1
  Product1/1 -> Demux/1
  Demux/1 -> Sum/1
  Demux/2 -> Sum/2
  Sum of Elements/1 -> Discrete Mean/1(In)
  Discrete Mean/1(Mean) -> P/1
  Sum/1 -> Discrete Mean1/1(In)
  Discrete Mean1/1(Mean) -> Q/1
  PLL (3ph)/1 -> Terminator/1

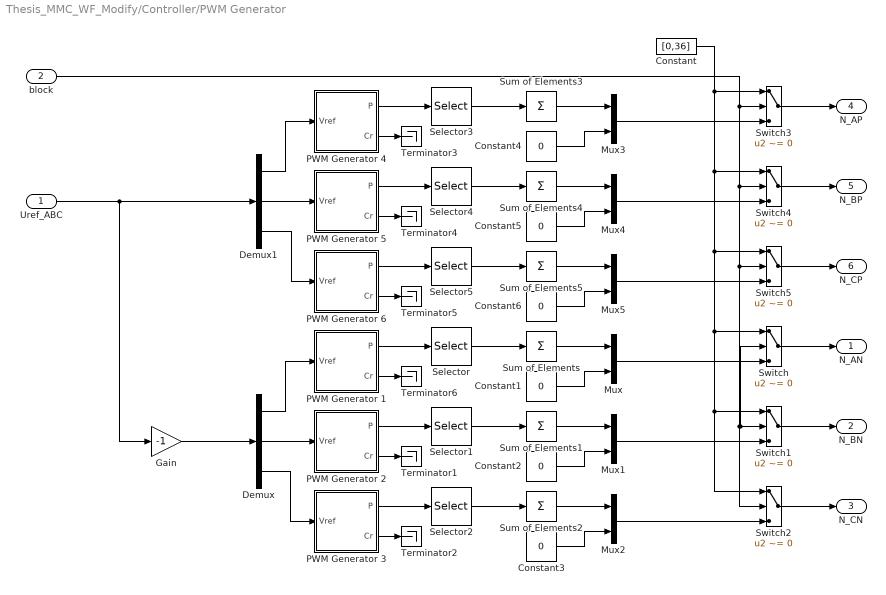
== system Thesis_MMC_WF_Modify/Controller/PWM Generator ==
  Uref_ABC : Inport
  block : Inport  Port=2
  Constant : Constant  Value=[0,36]
  Constant{1..6} (6 alike) : Constant  Value=0
  Demux : Demux  Outputs=3
  Demux1 : Demux  Outputs=3
  Gain : Gain  Gain=-1
  Mux{,1..5} (6 alike) : Mux  Inputs=2
  PWM Generator 1 : Subsystem
  PWM Generator 2 : Subsystem
  PWM Generator 3 : Subsystem
  PWM Generator 4 : Subsystem
  PWM Generator 5 : Subsystem
  PWM Generator 6 : Subsystem
  Selector{,1..5} (6 alike) : Selector  InputPortWidth=72  IndexOptions=Index vector (dialog)  Indices=[1:2:71]  OutputSizes=1
  Sum of Elements{,1..5} (6 alike) : Sum  Inputs=1
  Switch{,1..5} (6 alike) : Switch  Criteria=u2 ~= 0  SaturateOnIntegerOverflow=off  InputSameDT=off
  Terminator{1..6} (6 alike) : Terminator
  N_AN : Outport
  N_BN : Outport  Port=2
  N_CN : Outport  Port=3
  N_AP : Outport  Port=4
  N_BP : Outport  Port=5
  N_CP : Outport  Port=6
  wires:
  Switch/1 -> N_AN/1
  Switch1/1 -> N_BN/1
  Switch2/1 -> N_CN/1
  Switch3/1 -> N_AP/1
  Switch4/1 -> N_BP/1
  Switch5/1 -> N_CP/1
  block/1 -> Switch2/2, Switch/2, Switch1/2, Switch5/2, Switch4/2, Switch3/2
  Constant/1 -> Switch2/1, Switch1/1, Switch/1, Switch5/1, Switch4/1, Switch3/1
  PWM Generator 1/1(P) -> Selector/1
  Selector/1 -> Sum of Elements/1
  Sum of Elements/1 -> Mux/1
  Constant1/1 -> Mux/2
  Mux/1 -> Switch/3
  Demux/1 -> PWM Generator 1/1(Vref)
  PWM Generator 2/1(P) -> Selector1/1
  Selector1/1 -> Sum of Elements1/1
  Constant2/1 -> Mux1/2
  Sum of Elements1/1 -> Mux1/1
  PWM Generator 3/1(P) -> Selector2/1
  Selector2/1 -> Sum of Elements2/1
  Constant3/1 -> Mux2/2
  Sum of Elements2/1 -> Mux2/1
  Demux/2 -> PWM Generator 2/1(Vref)
  Demux/3 -> PWM Generator 3/1(Vref)
  Mux1/1 -> Switch1/3
  Mux2/1 -> Switch2/3
  PWM Generator 4/1(P) -> Selector3/1
  Selector3/1 -> Sum of Elements3/1
  Sum of Elements4/1 -> Mux4/1
  Constant4/1 -> Mux3/2
  Selector5/1 -> Sum of Elements5/1
  Sum of Elements3/1 -> Mux3/1
  Constant6/1 -> Mux5/2
  Selector4/1 -> Sum of Elements4/1
  Constant5/1 -> Mux4/2
  Sum of Elements5/1 -> Mux5/1
  PWM Generator 6/1(P) -> Selector5/1
  PWM Generator 5/1(P) -> Selector4/1
  Mux3/1 -> Switch3/3
  Mux4/1 -> Switch4/3
  Mux5/1 -> Switch5/3
  Demux1/2 -> PWM Generator 5/1(Vref)
  Demux1/1 -> PWM Generator 4/1(Vref)
  Demux1/3 -> PWM Generator 6/1(Vref)
  PWM Generator 2/2(Cr) -> Terminator1/1
  PWM Generator 3/2(Cr) -> Terminator2/1
  PWM Generator 4/2(Cr) -> Terminator3/1
  PWM Generator 5/2(Cr) -> Terminator4/1
  PWM Generator 6/2(Cr) -> Terminator5/1
  Uref_ABC/1 -> Gain/1, Demux1/1
  Gain/1 -> Demux/1
  PWM Generator 1/2(Cr) -> Terminator6/1

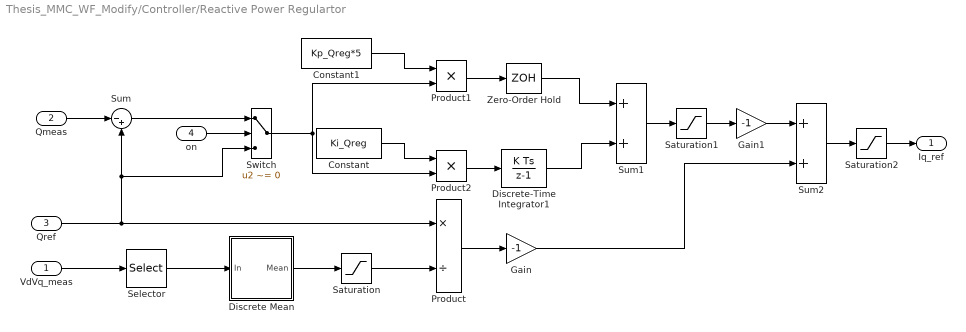
== system Thesis_MMC_WF_Modify/Controller/Reactive Power Regulartor ==
  VdVq_meas : Inport
  Qmeas : Inport  Port=2
  Qref : Inport  Port=3
  on : Inport  Port=4
  Constant : Constant  Value=Ki_Qreg
  Constant1 : Constant  Value=Kp_Qreg*5
  Discrete Mean : Subsystem
  Discrete-Time Integrator1 : DiscreteIntegrator  SampleTime=Ts_Control  LimitOutput=on  UpperSaturationLimit=Limits_Qreg(2)  LowerSaturationLimit=Limits_Qreg(1)  ICPrevOutput=DiscIntNeverNeededParam  ICPrevScaledInput=DiscIntNeverNeededParam
  Gain : Gain  Gain=-1
  Gain1 : Gain  Gain=-1
  Product : Product  Inputs=*/
  Product1 : Product
  Product2 : Product
  Saturation : Saturate  UpperLimit=2  LowerLimit=1e-6
  Saturation1 : Saturate  UpperLimit=Limits_Qreg(2)  LowerLimit=Limits_Qreg(1)
  Saturation2 : Saturate  UpperLimit=Limits_Qreg(2)  LowerLimit=Limits_Qreg(1)
  Selector : Selector  InputPortWidth=2  IndexOptions=Index vector (dialog)  Indices=[1]  OutputSizes=1
  Sum : Sum  Inputs=|-+
  Sum1 : Sum  SampleTime=Ts_Control
  Sum2 : Sum
  Switch : Switch  Criteria=u2 ~= 0  Threshold=0.5  SaturateOnIntegerOverflow=off  InputSameDT=off
  Zero-Order Hold : ZeroOrderHold  SampleTime=Ts_Control
  Iq_ref : Outport
  wires:
  VdVq_meas/1 -> Selector/1
  Saturation/1 -> Product/2
  Qref/1 -> Switch/3, Sum/2, Product/1
  on/1 -> Switch/2
  Sum/1 -> Switch/1
  Qmeas/1 -> Sum/1
  Product/1 -> Gain/1
  Switch/1 -> Product1/2, Product2/2
  Constant/1 -> Product2/1
  Constant1/1 -> Product1/1
  Product2/1 -> Discrete-Time Integrator1/1
  Product1/1 -> Zero-Order Hold/1
  Zero-Order Hold/1 -> Sum1/1
  Discrete-Time Integrator1/1 -> Sum1/2
  Sum1/1 -> Saturation1/1
  Saturation1/1 -> Gain1/1
  Gain1/1 -> Sum2/1
  Gain/1 -> Sum2/2
  Sum2/1 -> Saturation2/1
  Saturation2/1 -> Iq_ref/1
  Selector/1 -> Discrete Mean/1(In)
  Discrete Mean/1(Mean) -> Saturation/1

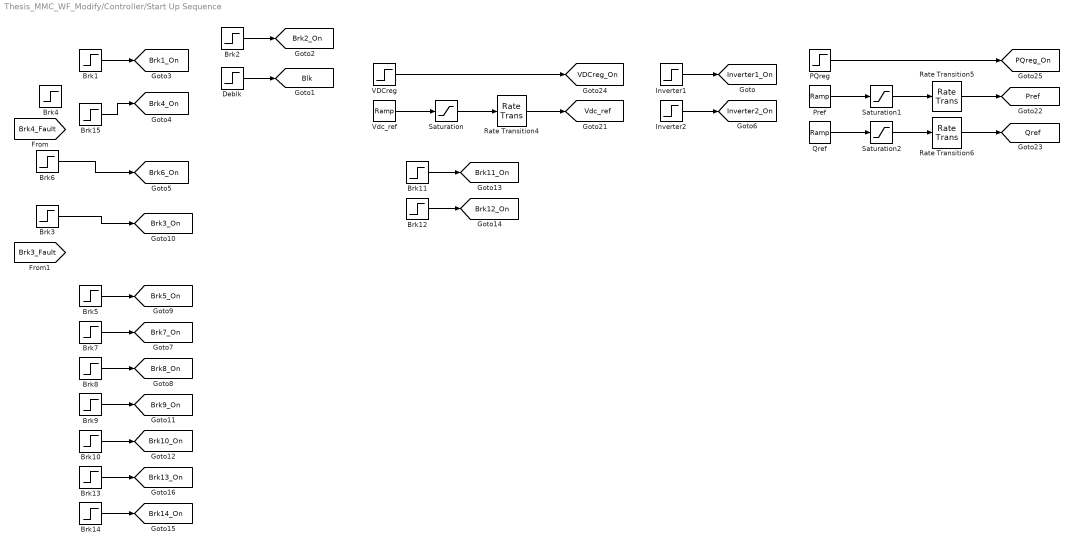
== system Thesis_MMC_WF_Modify/Controller/Start Up Sequence ==
  Brk1 : Step  Time=TBrk1_On  SampleTime=Ts_Power
  Brk{3..10,13..14} (10 alike) : Step  Time=0.1  SampleTime=Ts_Power
  Brk11 : Step  Time=7.48  SampleTime=Ts_Power
  Brk12 : Step  Time=7.48  SampleTime=Ts_Power
  Brk15 : Step  Time=10.3  Before=1  After=0  SampleTime=Ts_Power
  Brk2 : Step  Time=TBrk2_On  SampleTime=Ts_Power
  Deblk : Step  Time=1.5  Before=1  After=0  SampleTime=Ts_Power
  Inverter1 : Step  Time=4  SampleTime=Ts_Power
  Inverter2 : Step  Time=2.6  SampleTime=Ts_Power
  PQreg : Step  Time=Ton_PQreg  SampleTime=Ts_Control
  Pref : simulink/Sources/Ramp  slope=Slope_Pref  start=Tramping_Pref  InitialOutput=0
  Qref : simulink/Sources/Ramp  slope=-Slope_Qref*0.75  start=Tramping_Qref  InitialOutput=0
  Rate Transition4 : RateTransition  OutPortSampleTime=Ts_Control
  Rate Transition5 : RateTransition  OutPortSampleTime=Ts_Control
  Rate Transition6 : RateTransition  OutPortSampleTime=Ts_Control
  Saturation : Saturate  UpperLimit=Vnom_dc*52/64  LowerLimit=eps
  Saturation1 : Saturate  UpperLimit=1  LowerLimit=-1
  Saturation2 : Saturate  UpperLimit=Limits_Qreg(2)  LowerLimit=Limits_Qreg(1)
  VDCreg : Step  Time=Ton_VDCreg  SampleTime=Ts_Control
  Vdc_ref : simulink/Sources/Ramp  slope=Slope_Vdc_ref*0.9  start=Tramping_Vdc_ref  InitialOutput=Vnom_Sec*1.37*0.9
  tag scope: Blk=global, Brk10_On=global, Brk11_On=global, Brk12_On=global, Brk13_On=global, Brk14_On=global, Brk1_On=global, Brk2_On=global, Brk3_On=global, Brk4_On=global, Brk5_On=global, Brk6_On=global, Brk7_On=global, Brk8_On=global, Brk9_On=global, Inverter1_On=global, Inverter2_On=global, PQreg_On=global, Pref=global, Qref=global, VDCreg_On=global, Vdc_ref=global
  wires:
  Rate Transition4/1 -> [Vdc_ref]
  Rate Transition5/1 -> [Pref]
  Saturation/1 -> Rate Transition4/1
  Saturation1/1 -> Rate Transition5/1
  Pref/1 -> Saturation1/1
  VDCreg/1 -> [VDCreg_On]
  Saturation2/1 -> Rate Transition6/1
  Vdc_ref/1 -> Saturation/1
  PQreg/1 -> [PQreg_On]
  Inverter1/1 -> [Inverter1_On]
  Qref/1 -> Saturation2/1
  Rate Transition6/1 -> [Qref]
  Brk2/1 -> [Brk2_On]
  Brk1/1 -> [Brk1_On]
  Brk6/1 -> [Brk6_On]
  Inverter2/1 -> [Inverter2_On]
  Deblk/1 -> [Blk]
  Brk9/1 -> [Brk9_On]
  Brk8/1 -> [Brk8_On]
  Brk10/1 -> [Brk10_On]
  Brk7/1 -> [Brk7_On]
  Brk11/1 -> [Brk11_On]
  Brk12/1 -> [Brk12_On]
  Brk14/1 -> [Brk14_On]
  Brk13/1 -> [Brk13_On]
  Brk3/1 -> [Brk3_On]
  Brk5/1 -> [Brk5_On]
  Brk15/1 -> [Brk4_On]

== system Thesis_MMC_WF_Modify/MMC Converter/Filter A ==
  Breaker : spsBreakerLib/Breaker  InitialState=1  SwitchingTimes=Topen_Filter  External=off  BreakerResistance=0.001  SnubberResistance=1e6  SnubberCapacitance=inf  Measurements=None  MoreParameters=on  NoBreakLoop=off
  Current Measurement : spsCurrentMeasurementLib/Current Measurement  PhasorSimulation=off  OutputType=Complex  PSBequivalent=0
  Parallel RLC Branch : spsParallelRLCBranchLib/Parallel RLC Branch  LConnTagsString=a  RConnTagsString=__new0  BranchType=RC  Resistance=Rfilter  Inductance=1e-3  SetiL0=off  InitialCurrent=0  Capacitance=Cfilter  Setx0=off  InitialVoltage=0  Measurements=None
  Connection Port : PMIOPort  Side=Left
  Connection Port1 : PMIOPort  Port=2  Side=Left
  tag scope: FilterA=global
  wires:
  Current Measurement/1 -> [FilterA]
  connections:
  Parallel RLC Branch/RConn1 -- Connection Port/RConn1
  Current Measurement/RConn1 -- Parallel RLC Branch/LConn1
  Connection Port1/RConn1 -- Breaker/RConn1
  Breaker/LConn1 -- Current Measurement/LConn1

== system Thesis_MMC_WF_Modify/MMC Converter/Filter B ==
  Breaker : spsBreakerLib/Breaker  InitialState=1  SwitchingTimes=Topen_Filter  External=off  BreakerResistance=0.001  SnubberResistance=1e6  SnubberCapacitance=inf  Measurements=None  MoreParameters=on  NoBreakLoop=off
  Current Measurement : spsCurrentMeasurementLib/Current Measurement  PhasorSimulation=off  OutputType=Complex  PSBequivalent=0
  Parallel RLC Branch : spsParallelRLCBranchLib/Parallel RLC Branch  LConnTagsString=a  RConnTagsString=__new0  BranchType=RC  Resistance=Rfilter  Inductance=1e-3  SetiL0=off  InitialCurrent=0  Capacitance=Cfilter  Setx0=off  InitialVoltage=0  Measurements=None
  Connection Port : PMIOPort  Side=Left
  Connection Port1 : PMIOPort  Port=2  Side=Left
  tag scope: FilterB=global
  wires:
  Current Measurement/1 -> [FilterB]
  connections:
  Parallel RLC Branch/RConn1 -- Connection Port/RConn1
  Current Measurement/RConn1 -- Parallel RLC Branch/LConn1
  Connection Port1/RConn1 -- Breaker/RConn1
  Breaker/LConn1 -- Current Measurement/LConn1

== system Thesis_MMC_WF_Modify/MMC Converter/Filter C ==
  Breaker : spsBreakerLib/Breaker  InitialState=1  SwitchingTimes=Topen_Filter  External=off  BreakerResistance=0.001  SnubberResistance=1e6  SnubberCapacitance=inf  Measurements=None  MoreParameters=on  NoBreakLoop=off
  Current Measurement : spsCurrentMeasurementLib/Current Measurement  PhasorSimulation=off  OutputType=Complex  PSBequivalent=0
  Parallel RLC Branch : spsParallelRLCBranchLib/Parallel RLC Branch  LConnTagsString=a  RConnTagsString=__new0  BranchType=RC  Resistance=Rfilter  Inductance=1e-3  SetiL0=off  InitialCurrent=0  Capacitance=Cfilter  Setx0=off  InitialVoltage=0  Measurements=None
  Connection Port : PMIOPort  Side=Left
  Connection Port1 : PMIOPort  Port=2  Side=Left
  tag scope: FilterC=global
  wires:
  Current Measurement/1 -> [FilterC]
  connections:
  Parallel RLC Branch/RConn1 -- Connection Port/RConn1
  Current Measurement/RConn1 -- Parallel RLC Branch/LConn1
  Connection Port1/RConn1 -- Breaker/RConn1
  Breaker/LConn1 -- Current Measurement/LConn1

== system Thesis_MMC_WF_Modify/Controller/Current Regular/PI Regulator1 ==
  Error : Inport
  Compare To Zero : simulink/Logic and Bit Operations/Compare To Zero  relop=>  OutDataTypeStr=uint8  ZeroCross=off
  Compare To Zero1 : simulink/Logic and Bit Operations/Compare To Zero  relop=<  OutDataTypeStr=uint8  ZeroCross=off
  Constant : Constant  Value=UpperLimit
  Constant1 : Constant  Value=0
  Constant2 : Constant  Value=LowerLimit
  Discrete-Time Integrator : DiscreteIntegrator  IntegratorMethod=Integration: Trapezoidal  SampleTime=Ts_Control  LimitOutput=on  UpperSaturationLimit=UpperLimit  LowerSaturationLimit=LowerLimit  ShowStatePort=on  ICPrevOutput=DiscIntNeverNeededParam  ICPrevScaledInput=DiscIntNeverNeededParam
  Gain1 : Gain  SampleTime=Ts_Control
  Gain2 : Gain  Gain=Ki  SampleTime=Ts_Control
  Logical Operator : Logic  AllPortsSameDT=off  OutDataTypeStr=boolean
  Logical Operator1 : Logic  Operator=OR  AllPortsSameDT=off  OutDataTypeStr=boolean
  Logical Operator2 : Logic  AllPortsSameDT=off  OutDataTypeStr=boolean
  Relational Operator : RelationalOperator  Operator=<=  OutDataTypeStr=boolean  RndMeth=Simplest  InputSameDT=off
  Relational Operator1 : RelationalOperator  OutDataTypeStr=boolean  RndMeth=Simplest  InputSameDT=off
  Saturation : Saturate  UpperLimit=UpperLimit  LowerLimit=LowerLimit  SampleTime=Ts_Control
  Sum1 : Sum  SampleTime=Ts_Control
  Sum2 : Sum  SampleTime=Ts_Control
  Switch : Switch  Criteria=u2 > Threshold  SaturateOnIntegerOverflow=off  InputSameDT=off
  Zero-Order Hold : ZeroOrderHold  SampleTime=Ts_Control
  Out : Outport
  wires:
  Constant1/1 -> Switch/1
  Gain2/1 -> Switch/3
  Gain1/1 -> Zero-Order Hold/1
  Error/1 -> Compare To Zero1/1, Compare To Zero/1, Gain2/1, Gain1/1
  Switch/1 -> Discrete-Time Integrator/1
  Zero-Order Hold/1 -> Sum2/2, Sum1/1
  Saturation/1 -> Out/1
  Sum2/1 -> Relational Operator/1, Relational Operator1/1
  Discrete-Time Integrator/State -> Sum2/1
  Constant/1 -> Relational Operator1/2
  Constant2/1 -> Relational Operator/2
  Logical Operator1/1 -> Switch/2
  Compare To Zero/1 -> Logical Operator/2
  Compare To Zero1/1 -> Logical Operator2/2
  Relational Operator1/1 -> Logical Operator/1
  Relational Operator/1 -> Logical Operator2/1
  Logical Operator2/1 -> Logical Operator1/1
  Logical Operator/1 -> Logical Operator1/2
  Sum1/1 -> Saturation/1
  Discrete-Time Integrator/1 -> Sum1/2
